simulink library "halin"  (R2021b)
settings: Solver=VariableStepAuto  StartTime=0.0  StopTime=10.0  RelTol=1e-3
undefined symbols (not defined in the file): KHAL_CAN1ABM1E2E_flg, KHAL_CAN1EPB1E2E_flg, KHAL_CAN1EPS1E2E_flg, KHAL_CAN1ESC1E2E_flg, KHAL_CAN1ESC5E2E_flg, KHAL_CAN3BMS1E2E_flg, KHAL_CAN3BMS6E2E_flg, KHAL_CAN3CCU1E2E_flg, KHAL_CAN3CCU2E2E_flg, KHAL_CAN3MCUBF1E2E_flg, KHAL_CAN3MCUBR1E2E_flg, KHAL_CAN3MCUNF1E2E_flg, KHAL_CAN3MCUNR1E2E_flg, KHAL_CAN3Shifter1E2E_flg, KHAL_CAN3Shifter2E2E_flg, KHAL_CAN6FCM2E2E_flg, KHAL_CAN6FCM4E2E_flg, TRUE
libraries: simulink x791, FVT_lib x214, hcu_lib x58
(part 14 of 25)

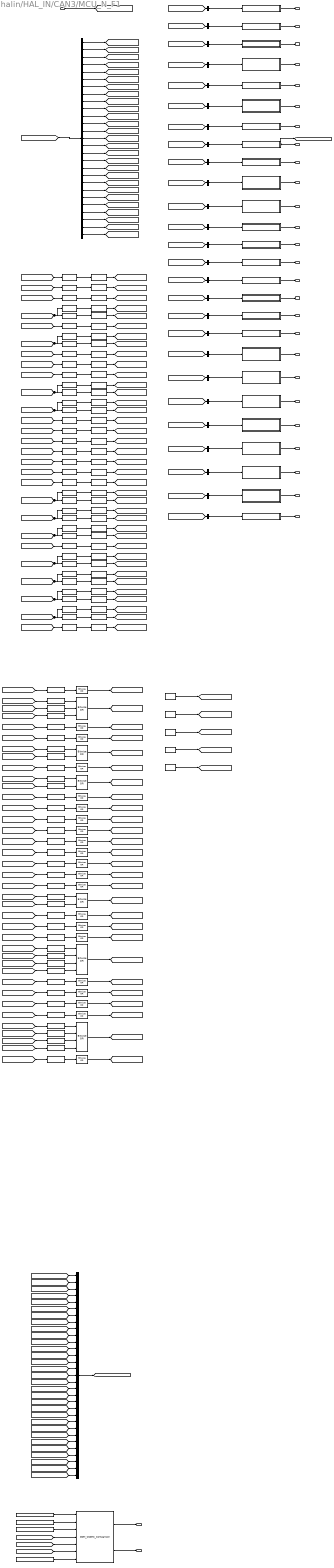
== system halin/HAL_IN/CAN3/MCU_N_F1 ==
  DT_CAN3_SG_MCU_N_F1 : Inport
  0x95 : Constant  Value=0x95
  0xF9 : Constant  Value=0xF9
  BitwiseAND{,1..37} (38 alike) : simulink/Logic and Bit Operations/Bitwise Operator  logicop=AND  UseBitMask=on  BitMask=0xFF  BitMaskRealWorld=Stored Integer
  BitwiseOR{,2..3,5,7..15,17..19,21..24,26} (21 alike) : simulink/Logic and Bit Operations/Bitwise Operator  logicop=OR  UseBitMask=off  BitMask=bin2dec('11011001')  BitMaskRealWorld=Stored Integer
  BitwiseOR1 : simulink/Logic and Bit Operations/Bitwise Operator  logicop=OR  UseBitMask=off  NumInputPorts=3  BitMask=bin2dec('11011001')  BitMaskRealWorld=Stored Integer
  BitwiseOR16 : simulink/Logic and Bit Operations/Bitwise Operator  logicop=OR  UseBitMask=off  NumInputPorts=2  BitMask=bin2dec('11011001')  BitMaskRealWorld=Stored Integer
  BitwiseOR20 : simulink/Logic and Bit Operations/Bitwise Operator  logicop=OR  UseBitMask=off  NumInputPorts=4  BitMask=bin2dec('11011001')  BitMaskRealWorld=Stored Integer
  BitwiseOR25 : simulink/Logic and Bit Operations/Bitwise Operator  logicop=OR  UseBitMask=off  NumInputPorts=4  BitMask=bin2dec('11011001')  BitMaskRealWorld=Stored Integer
  BitwiseOR4 : simulink/Logic and Bit Operations/Bitwise Operator  logicop=OR  UseBitMask=off  NumInputPorts=2  BitMask=bin2dec('11011001')  BitMaskRealWorld=Stored Integer
  BitwiseOR6 : simulink/Logic and Bit Operations/Bitwise Operator  logicop=OR  UseBitMask=off  NumInputPorts=2  BitMask=bin2dec('11011001')  BitMaskRealWorld=Stored Integer
  DDM_CS&RC_Comparison : FVT_lib/hal/DDM_CS&RC_Comparison  MsgCycleTime=100
  Data Type Conversion{,1..37} (38 alike) : DataTypeConversion  OutDataTypeStr=uint8
  FrActvDmpDisabStaNidec : Subsystem
  FrEDUDrtStaNidec : Subsystem
  FrEDUOpratingStaNidec : Subsystem
  FrEDURealTMTqNidec : Subsystem
  FrEDURotateDirctionNidec : Subsystem
  FrEDUTqReqFbkNidec : Subsystem
  FrMCU1ChksumNidec : Subsystem
  FrMCU1RolCntNidec : Subsystem
  FrMCUBATNidec : Subsystem
  FrMCUDCBusCurrNidec : Subsystem
  FrMCUDCBusVoltNidec : Subsystem
  FrMCUDischrgStaNidec : Subsystem
  FrMCUEnaStaNidec : Subsystem
  FrMCUErrNidec : Subsystem
  FrMCUIGNstaNidec : Subsystem
  FrMCUReady4PreNidec : Subsystem
  FrMCUReadyNidec : Subsystem
  FrMCUSysStaNidec : Subsystem
  FrMCUTempNidec : Subsystem
  FrMotorAvailTqNidec : Subsystem
  FrRegenAvailTqNidec : Subsystem
  FrTMSpdNidec : Subsystem
  FrTMTempNidec : Subsystem
  FrTMidNidec : Subsystem
  FrTMiqNidec : Subsystem
  KHAL_CAN3MCUNF1E2E_flg : Constant  Value=KHAL_CAN3MCUNF1E2E_flg
  LeftShift : ArithShift  BitShiftNumber=1  BitShiftDirection=Left
  LeftShift1 : ArithShift  BitShiftNumber=2  BitShiftDirection=Left
  LeftShift{4,6,9..11,13,15} (7 alike) : ArithShift  BitShiftDirection=Left
  LeftShift12 : ArithShift  BitShiftNumber=3  BitShiftDirection=Left
  LeftShift14 : ArithShift  BitShiftNumber=1  BitShiftDirection=Left
  LeftShift2 : ArithShift  BitShiftNumber=5  BitShiftDirection=Left
  LeftShift3 : ArithShift  BitShiftNumber=6  BitShiftDirection=Left
  LeftShift5 : ArithShift  BitShiftNumber=4  BitShiftDirection=Left
  LeftShift7 : ArithShift  BitShiftNumber=3  BitShiftDirection=Left
  LeftShift8 : ArithShift  BitShiftNumber=4  BitShiftDirection=Left
  MCUWarnFNidec : Subsystem
  MessageRollingCounter : FVT_lib/hal/MessageRollingCounter  CounterMAX=14  task_time_ms=5  msg_time_ms=100
  Mux : Mux  Inputs=31
  RightShift{,2,4,6,10,14,16,18,20} (9 alike) : ArithShift  BitShiftNumber=8
  RightShift{1,3,5,7,11,15,17,19,21} (9 alike) : ArithShift
  RightShift12 : ArithShift  BitShiftNumber=4
  RightShift13 : ArithShift  BitShiftNumber=-4
  RightShift8 : ArithShift  BitShiftNumber=1
  RightShift9 : ArithShift  BitShiftNumber=-7
  bus_selector : BusSelector  OutputSignals=CAN3_Fr_ActvDmpDisabSta_Nidec,CAN3_Fr_EDUDrtSta_Nidec,CAN3_Fr_EDUOpratingSta_Nidec,CAN3_Fr_EDURealTMTq_Nidec,CAN3_Fr_EDURotateDirction_Nidec,CAN3_Fr_EDUTqReqFbk_Nidec,CAN3_Fr_MCU1Chksum_Nidec,CAN3_Fr_MCU1RolCnt_Nidec,CAN3_Fr_MCUBAT_Nidec,CAN3_Fr_MCUDCBusCurr_Nidec,CAN3_Fr_MCUDCBusVolt_Nidec,CAN3_Fr_MCUDischrgSta_Nidec,CAN3_Fr_MCUEnaSta_Nidec,CAN3_Fr_MCUErr_Nidec,CAN3_Fr_MCUIGN_sta_Nidec,CAN3_Fr_MCUReady4Pre_Nidec,CAN3_Fr_MCUReady_Nidec,CAN3_Fr_MCUSysSta_Nidec,CAN3_Fr_MCUTemp_Nidec,CAN3_Fr_MotorAvailTq_Nidec,CAN3_Fr_RegenAvailTq_Nidec,CAN3_Fr_Reserved_bits_Nidec,CAN3_Fr_TMSpd_Nidec,CAN3_Fr_TMTemp_Nidec,CAN3_Fr_TMid_Nidec,CAN3_Fr_TMiq_Nidec,CAN3_MCUWarn_F_Nidec
  bus_selector1 : BusSelector  OutputSignals=CAN3_Fr_ActvDmpDisabSta_Nidec
  bus_selector10 : BusSelector  OutputSignals=CAN3_Fr_MCUDCBusCurr_Nidec
  bus_selector11 : BusSelector  OutputSignals=CAN3_Fr_MCUDCBusVolt_Nidec
  bus_selector12 : BusSelector  OutputSignals=CAN3_Fr_MCUDischrgSta_Nidec
  bus_selector13 : BusSelector  OutputSignals=CAN3_Fr_MCUEnaSta_Nidec
  bus_selector14 : BusSelector  OutputSignals=CAN3_Fr_MCUErr_Nidec
  bus_selector15 : BusSelector  OutputSignals=CAN3_Fr_MCUIGN_sta_Nidec
  bus_selector16 : BusSelector  OutputSignals=CAN3_Fr_MCUReady4Pre_Nidec
  bus_selector17 : BusSelector  OutputSignals=CAN3_Fr_MCUReady_Nidec
  bus_selector18 : BusSelector  OutputSignals=CAN3_Fr_MCUSysSta_Nidec
  bus_selector19 : BusSelector  OutputSignals=CAN3_Fr_MCUTemp_Nidec
  bus_selector2 : BusSelector  OutputSignals=CAN3_Fr_EDUDrtSta_Nidec
  bus_selector20 : BusSelector  OutputSignals=CAN3_Fr_MotorAvailTq_Nidec
  bus_selector21 : BusSelector  OutputSignals=CAN3_Fr_RegenAvailTq_Nidec
  bus_selector22 : BusSelector  OutputSignals=CAN3_Fr_TMSpd_Nidec
  bus_selector23 : BusSelector  OutputSignals=CAN3_Fr_TMTemp_Nidec
  bus_selector24 : BusSelector  OutputSignals=CAN3_Fr_TMid_Nidec
  bus_selector25 : BusSelector  OutputSignals=CAN3_Fr_TMiq_Nidec
  bus_selector26 : BusSelector  OutputSignals=CAN3_MCUWarn_F_Nidec
  bus_selector3 : BusSelector  OutputSignals=CAN3_Fr_EDUOpratingSta_Nidec
  bus_selector4 : BusSelector  OutputSignals=CAN3_Fr_EDURealTMTq_Nidec
  bus_selector5 : BusSelector  OutputSignals=CAN3_Fr_EDURotateDirction_Nidec
  bus_selector6 : BusSelector  OutputSignals=CAN3_Fr_EDUTqReqFbk_Nidec
  bus_selector7 : BusSelector  OutputSignals=CAN3_Fr_MCU1Chksum_Nidec
  bus_selector8 : BusSelector  OutputSignals=CAN3_Fr_MCU1RolCnt_Nidec
  bus_selector9 : BusSelector  OutputSignals=CAN3_Fr_MCUBAT_Nidec
  constant{,1..4} (5 alike) : Constant  Value=0x0  OutDataTypeStr=uint8
  VHAL_MCUNF1CSErr_flg : Outport
  VHAL_MCUNF1RCErr_flg : Outport  Port=2
  VHAL_FrActvDmpDisabStaNidec_flg : Outport  Port=3
  VHAL_FrEDUDrtStaNidec_flg : Outport  Port=4
  VHAL_FrEDUOpratingStaNidec_flg : Outport  Port=5
  VHAL_FrEDURealTMTqNidec_Nm : Outport  Port=6
  VHAL_FrEDURotateDirctionNidec_enum : Outport  Port=7
  VHAL_FrEDUTqReqFbkNidec_Nm : Outport  Port=8
  VHAL_FrMCU1ChksumNidec_enum : Outport  Port=9
  VHAL_FrMCU1RolCntNidec_enum : Outport  Port=10
  VHAL_FrMCUBATNidec_V : Outport  Port=11
  VHAL_FrMCUDCBusCurrNidec_A : Outport  Port=12
  VHAL_FrMCUDCBusVoltNidec_V : Outport  Port=13
  VHAL_FrMCUDischrgStaNidec_flg : Outport  Port=14
  VHAL_FrMCUEnaStaNidec_flg : Outport  Port=15
  VHAL_FrMCUErrNidec_enum : Outport  Port=16
  VHAL_FrMCUIGNstaNidec_flg : Outport  Port=17
  VHAL_FrMCUReady4PreNidec_flg : Outport  Port=18
  VHAL_FrMCUReadyNidec_flg : Outport  Port=19
  VHAL_FrMCUSysStaNidec_enum : Outport  Port=20
  VHAL_FrMCUTempNidec_C : Outport  Port=21
  VHAL_FrMotorAvailTqNidec_Nm : Outport  Port=22
  VHAL_FrRegenAvailTqNidec_Nm : Outport  Port=23
  VHAL_FrTMSpdNidec_rpm : Outport  Port=24
  VHAL_FrTMTempNidec_C : Outport  Port=25
  VHAL_FrTMidNidec_A : Outport  Port=26
  VHAL_FrTMiqNidec_A : Outport  Port=27
  VHAL_MCUWarnFNidec_enum : Outport  Port=28
  wires:
  DT_CAN3_SG_MCU_N_F1/1 -> [DT_CAN3_SG_MCU_N_F1]
  [DT_CAN3_SG_MCU_N_F1] -> bus_selector/1
  bus_selector/1 -> [CAN3_Fr_ActvDmpDisabSta_Nidec]  "<CAN3_Fr_ActvDmpDisabSta_Nidec>"
  [CAN3_Fr_ActvDmpDisabSta_Nidec] -> LeftShift/1
  LeftShift/1 -> BitwiseAND/1
  BitwiseAND/1 -> [Byte_25_CAN3_Fr_ActvDmpDisabSta_Nidec]
  bus_selector/2 -> [CAN3_Fr_EDUDrtSta_Nidec]  "<CAN3_Fr_EDUDrtSta_Nidec>"
  [CAN3_Fr_EDUDrtSta_Nidec] -> LeftShift1/1
  LeftShift1/1 -> BitwiseAND1/1
  BitwiseAND1/1 -> [Byte_25_CAN3_Fr_EDUDrtSta_Nidec]
  bus_selector/3 -> [CAN3_Fr_EDUOpratingSta_Nidec]  "<CAN3_Fr_EDUOpratingSta_Nidec>"
  [CAN3_Fr_EDUOpratingSta_Nidec] -> LeftShift2/1
  LeftShift2/1 -> BitwiseAND2/1
  BitwiseAND2/1 -> [Byte_30_CAN3_Fr_EDUOpratingSta_Nidec]
  bus_selector/4 -> [CAN3_Fr_EDURealTMTq_Nidec]  "<CAN3_Fr_EDURealTMTq_Nidec>"
  [CAN3_Fr_EDURealTMTq_Nidec] -> RightShift/1, RightShift1/1
  RightShift/1 -> BitwiseAND3/1
  BitwiseAND3/1 -> [Byte_28_CAN3_Fr_EDURealTMTq_Nidec]
  RightShift1/1 -> BitwiseAND4/1
  BitwiseAND4/1 -> [Byte_29_CAN3_Fr_EDURealTMTq_Nidec]
  bus_selector/5 -> [CAN3_Fr_EDURotateDirction_Nidec]  "<CAN3_Fr_EDURotateDirction_Nidec>"
  [CAN3_Fr_EDURotateDirction_Nidec] -> LeftShift3/1
  LeftShift3/1 -> BitwiseAND5/1
  BitwiseAND5/1 -> [Byte_30_CAN3_Fr_EDURotateDirction_Nidec]
  bus_selector/6 -> [CAN3_Fr_EDUTqReqFbk_Nidec]  "<CAN3_Fr_EDUTqReqFbk_Nidec>"
  [CAN3_Fr_EDUTqReqFbk_Nidec] -> RightShift2/1, RightShift3/1
  RightShift2/1 -> BitwiseAND6/1
  BitwiseAND6/1 -> [Byte_30_CAN3_Fr_EDUTqReqFbk_Nidec]
  RightShift3/1 -> BitwiseAND7/1
  BitwiseAND7/1 -> [Byte_31_CAN3_Fr_EDUTqReqFbk_Nidec]
  bus_selector/7 -> [CAN3_Fr_MCU1Chksum_Nidec]  "<CAN3_Fr_MCU1Chksum_Nidec>"
  [CAN3_Fr_MCU1Chksum_Nidec] -> LeftShift4/1
  LeftShift4/1 -> BitwiseAND8/1
  BitwiseAND8/1 -> [Byte_0_CAN3_Fr_MCU1Chksum_Nidec]
  bus_selector/8 -> [CAN3_Fr_MCU1RolCnt_Nidec]  "<CAN3_Fr_MCU1RolCnt_Nidec>"
  [CAN3_Fr_MCU1RolCnt_Nidec] -> LeftShift5/1
  LeftShift5/1 -> BitwiseAND9/1
  BitwiseAND9/1 -> [Byte_1_CAN3_Fr_MCU1RolCnt_Nidec]
  bus_selector/9 -> [CAN3_Fr_MCUBAT_Nidec]  "<CAN3_Fr_MCUBAT_Nidec>"
  [CAN3_Fr_MCUBAT_Nidec] -> LeftShift6/1
  LeftShift6/1 -> BitwiseAND10/1
  BitwiseAND10/1 -> [Byte_8_CAN3_Fr_MCUBAT_Nidec]
  bus_selector/10 -> [CAN3_Fr_MCUDCBusCurr_Nidec]  "<CAN3_Fr_MCUDCBusCurr_Nidec>"
  [CAN3_Fr_MCUDCBusCurr_Nidec] -> RightShift4/1, RightShift5/1
  RightShift4/1 -> BitwiseAND11/1
  BitwiseAND11/1 -> [Byte_21_CAN3_Fr_MCUDCBusCurr_Nidec]
  RightShift5/1 -> BitwiseAND12/1
  BitwiseAND12/1 -> [Byte_22_CAN3_Fr_MCUDCBusCurr_Nidec]
  bus_selector/11 -> [CAN3_Fr_MCUDCBusVolt_Nidec]  "<CAN3_Fr_MCUDCBusVolt_Nidec>"
  [CAN3_Fr_MCUDCBusVolt_Nidec] -> RightShift6/1, RightShift7/1
  RightShift6/1 -> BitwiseAND13/1
  BitwiseAND13/1 -> [Byte_23_CAN3_Fr_MCUDCBusVolt_Nidec]
  RightShift7/1 -> BitwiseAND14/1
  BitwiseAND14/1 -> [Byte_24_CAN3_Fr_MCUDCBusVolt_Nidec]
  bus_selector/12 -> [CAN3_Fr_MCUDischrgSta_Nidec]  "<CAN3_Fr_MCUDischrgSta_Nidec>"
  [CAN3_Fr_MCUDischrgSta_Nidec] -> LeftShift7/1
  LeftShift7/1 -> BitwiseAND15/1
  BitwiseAND15/1 -> [Byte_25_CAN3_Fr_MCUDischrgSta_Nidec]
  bus_selector/13 -> [CAN3_Fr_MCUEnaSta_Nidec]  "<CAN3_Fr_MCUEnaSta_Nidec>"
  [CAN3_Fr_MCUEnaSta_Nidec] -> LeftShift8/1
  LeftShift8/1 -> BitwiseAND16/1
  BitwiseAND16/1 -> [Byte_30_CAN3_Fr_MCUEnaSta_Nidec]
  bus_selector/14 -> [CAN3_Fr_MCUErr_Nidec]  "<CAN3_Fr_MCUErr_Nidec>"
  [CAN3_Fr_MCUErr_Nidec] -> LeftShift9/1
  LeftShift9/1 -> BitwiseAND17/1
  BitwiseAND17/1 -> [Byte_17_CAN3_Fr_MCUErr_Nidec]
  bus_selector/15 -> [CAN3_Fr_MCUIGN_sta_Nidec]  "<CAN3_Fr_MCUIGN_sta_Nidec>"
  [CAN3_Fr_MCUIGN_sta_Nidec] -> LeftShift10/1
  LeftShift10/1 -> BitwiseAND18/1
  BitwiseAND18/1 -> [Byte_9_CAN3_Fr_MCUIGN_sta_Nidec]
  bus_selector/16 -> [CAN3_Fr_MCUReady4Pre_Nidec]  "<CAN3_Fr_MCUReady4Pre_Nidec>"
  [CAN3_Fr_MCUReady4Pre_Nidec] -> LeftShift11/1
  LeftShift11/1 -> BitwiseAND19/1
  BitwiseAND19/1 -> [Byte_25_CAN3_Fr_MCUReady4Pre_Nidec]
  bus_selector/17 -> [CAN3_Fr_MCUReady_Nidec]  "<CAN3_Fr_MCUReady_Nidec>"
  [CAN3_Fr_MCUReady_Nidec] -> LeftShift12/1
  LeftShift12/1 -> BitwiseAND20/1
  BitwiseAND20/1 -> [Byte_1_CAN3_Fr_MCUReady_Nidec]
  bus_selector/18 -> [CAN3_Fr_MCUSysSta_Nidec]  "<CAN3_Fr_MCUSysSta_Nidec>"
  [CAN3_Fr_MCUSysSta_Nidec] -> LeftShift13/1
  LeftShift13/1 -> BitwiseAND21/1
  BitwiseAND21/1 -> [Byte_7_CAN3_Fr_MCUSysSta_Nidec]
  bus_selector/19 -> [CAN3_Fr_MCUTemp_Nidec]  "<CAN3_Fr_MCUTemp_Nidec>"
  [CAN3_Fr_MCUTemp_Nidec] -> RightShift8/1, RightShift9/1
  RightShift8/1 -> BitwiseAND22/1
  BitwiseAND22/1 -> [Byte_20_CAN3_Fr_MCUTemp_Nidec]
  RightShift9/1 -> BitwiseAND23/1
  BitwiseAND23/1 -> [Byte_21_CAN3_Fr_MCUTemp_Nidec]
  bus_selector/20 -> [CAN3_Fr_MotorAvailTq_Nidec]  "<CAN3_Fr_MotorAvailTq_Nidec>"
  [CAN3_Fr_MotorAvailTq_Nidec] -> RightShift10/1, RightShift11/1
  RightShift10/1 -> BitwiseAND24/1
  BitwiseAND24/1 -> [Byte_11_CAN3_Fr_MotorAvailTq_Nidec]
  RightShift11/1 -> BitwiseAND25/1
  BitwiseAND25/1 -> [Byte_12_CAN3_Fr_MotorAvailTq_Nidec]
  bus_selector/21 -> [CAN3_Fr_RegenAvailTq_Nidec]  "<CAN3_Fr_RegenAvailTq_Nidec>"
  [CAN3_Fr_RegenAvailTq_Nidec] -> RightShift12/1, RightShift13/1
  RightShift12/1 -> BitwiseAND26/1
  BitwiseAND26/1 -> [Byte_10_CAN3_Fr_RegenAvailTq_Nidec]
  RightShift13/1 -> BitwiseAND27/1
  BitwiseAND27/1 -> [Byte_11_CAN3_Fr_RegenAvailTq_Nidec]
  bus_selector/22 -> [CAN3_Fr_Reserved_bits_Nidec]  "<CAN3_Fr_Reserved_bits_Nidec>"
  [CAN3_Fr_Reserved_bits_Nidec] -> LeftShift14/1
  LeftShift14/1 -> BitwiseAND28/1
  BitwiseAND28/1 -> [Byte_9_CAN3_Fr_Reserved_bits_Nidec]
  bus_selector/23 -> [CAN3_Fr_TMSpd_Nidec]  "<CAN3_Fr_TMSpd_Nidec>"
  [CAN3_Fr_TMSpd_Nidec] -> RightShift14/1, RightShift15/1
  RightShift14/1 -> BitwiseAND29/1
  BitwiseAND29/1 -> [Byte_26_CAN3_Fr_TMSpd_Nidec]
  RightShift15/1 -> BitwiseAND30/1
  BitwiseAND30/1 -> [Byte_27_CAN3_Fr_TMSpd_Nidec]
  bus_selector/24 -> [CAN3_Fr_TMTemp_Nidec]  "<CAN3_Fr_TMTemp_Nidec>"
  [CAN3_Fr_TMTemp_Nidec] -> RightShift16/1, RightShift17/1
  RightShift16/1 -> BitwiseAND31/1
  BitwiseAND31/1 -> [Byte_18_CAN3_Fr_TMTemp_Nidec]
  RightShift17/1 -> BitwiseAND32/1
  BitwiseAND32/1 -> [Byte_19_CAN3_Fr_TMTemp_Nidec]
  bus_selector/25 -> [CAN3_Fr_TMid_Nidec]  "<CAN3_Fr_TMid_Nidec>"
  [CAN3_Fr_TMid_Nidec] -> RightShift18/1, RightShift19/1
  RightShift18/1 -> BitwiseAND33/1
  BitwiseAND33/1 -> [Byte_15_CAN3_Fr_TMid_Nidec]
  RightShift19/1 -> BitwiseAND34/1
  BitwiseAND34/1 -> [Byte_16_CAN3_Fr_TMid_Nidec]
  bus_selector/26 -> [CAN3_Fr_TMiq_Nidec]  "<CAN3_Fr_TMiq_Nidec>"
  [CAN3_Fr_TMiq_Nidec] -> RightShift20/1, RightShift21/1
  RightShift20/1 -> BitwiseAND35/1
  BitwiseAND35/1 -> [Byte_13_CAN3_Fr_TMiq_Nidec]
  RightShift21/1 -> BitwiseAND36/1
  BitwiseAND36/1 -> [Byte_14_CAN3_Fr_TMiq_Nidec]
  bus_selector/27 -> [CAN3_MCUWarn_F_Nidec]  "<CAN3_MCUWarn_F_Nidec>"
  [CAN3_MCUWarn_F_Nidec] -> LeftShift15/1
  LeftShift15/1 -> BitwiseAND37/1
  BitwiseAND37/1 -> [Byte_1_CAN3_MCUWarn_F_Nidec]
  Data Type Conversion/1 -> BitwiseOR/1
  [Byte_0_CAN3_Fr_MCU1Chksum_Nidec] -> Data Type Conversion/1
  BitwiseOR/1 -> [Byte_0]
  Data Type Conversion1/1 -> BitwiseOR1/1
  [Byte_1_CAN3_Fr_MCU1RolCnt_Nidec] -> Data Type Conversion1/1
  Data Type Conversion2/1 -> BitwiseOR1/2
  [Byte_1_CAN3_Fr_MCUReady_Nidec] -> Data Type Conversion2/1
  Data Type Conversion3/1 -> BitwiseOR1/3
  [Byte_1_CAN3_MCUWarn_F_Nidec] -> Data Type Conversion3/1
  BitwiseOR1/1 -> [Byte_1]
  constant/1 -> [Byte_2]
  constant1/1 -> [Byte_3]
  constant2/1 -> [Byte_4]
  constant3/1 -> [Byte_5]
  constant4/1 -> [Byte_6]
  Data Type Conversion4/1 -> BitwiseOR2/1
  [Byte_7_CAN3_Fr_MCUSysSta_Nidec] -> Data Type Conversion4/1
  BitwiseOR2/1 -> [Byte_7]
  Data Type Conversion5/1 -> BitwiseOR3/1
  [Byte_8_CAN3_Fr_MCUBAT_Nidec] -> Data Type Conversion5/1
  BitwiseOR3/1 -> [Byte_8]
  Data Type Conversion6/1 -> BitwiseOR4/1
  [Byte_9_CAN3_Fr_MCUIGN_sta_Nidec] -> Data Type Conversion6/1
  Data Type Conversion7/1 -> BitwiseOR4/2
  [Byte_9_CAN3_Fr_Reserved_bits_Nidec] -> Data Type Conversion7/1
  BitwiseOR4/1 -> [Byte_9]
  Data Type Conversion8/1 -> BitwiseOR5/1
  [Byte_10_CAN3_Fr_RegenAvailTq_Nidec] -> Data Type Conversion8/1
  BitwiseOR5/1 -> [Byte_10]
  Data Type Conversion9/1 -> BitwiseOR6/1
  [Byte_11_CAN3_Fr_MotorAvailTq_Nidec] -> Data Type Conversion9/1
  Data Type Conversion10/1 -> BitwiseOR6/2
  [Byte_11_CAN3_Fr_RegenAvailTq_Nidec] -> Data Type Conversion10/1
  BitwiseOR6/1 -> [Byte_11]
  Data Type Conversion11/1 -> BitwiseOR7/1
  [Byte_12_CAN3_Fr_MotorAvailTq_Nidec] -> Data Type Conversion11/1
  BitwiseOR7/1 -> [Byte_12]
  Data Type Conversion12/1 -> BitwiseOR8/1
  [Byte_13_CAN3_Fr_TMiq_Nidec] -> Data Type Conversion12/1
  BitwiseOR8/1 -> [Byte_13]
  Data Type Conversion13/1 -> BitwiseOR9/1
  [Byte_14_CAN3_Fr_TMiq_Nidec] -> Data Type Conversion13/1
  BitwiseOR9/1 -> [Byte_14]
  Data Type Conversion14/1 -> BitwiseOR10/1
  [Byte_15_CAN3_Fr_TMid_Nidec] -> Data Type Conversion14/1
  BitwiseOR10/1 -> [Byte_15]
  Data Type Conversion15/1 -> BitwiseOR11/1
  [Byte_16_CAN3_Fr_TMid_Nidec] -> Data Type Conversion15/1
  BitwiseOR11/1 -> [Byte_16]
  Data Type Conversion16/1 -> BitwiseOR12/1
  [Byte_17_CAN3_Fr_MCUErr_Nidec] -> Data Type Conversion16/1
  BitwiseOR12/1 -> [Byte_17]
  Data Type Conversion17/1 -> BitwiseOR13/1
  [Byte_18_CAN3_Fr_TMTemp_Nidec] -> Data Type Conversion17/1
  BitwiseOR13/1 -> [Byte_18]
  Data Type Conversion18/1 -> BitwiseOR14/1
  [Byte_19_CAN3_Fr_TMTemp_Nidec] -> Data Type Conversion18/1
  BitwiseOR14/1 -> [Byte_19]
  Data Type Conversion19/1 -> BitwiseOR15/1
  [Byte_20_CAN3_Fr_MCUTemp_Nidec] -> Data Type Conversion19/1
  BitwiseOR15/1 -> [Byte_20]
  Data Type Conversion20/1 -> BitwiseOR16/1
  [Byte_21_CAN3_Fr_MCUDCBusCurr_Nidec] -> Data Type Conversion20/1
  Data Type Conversion21/1 -> BitwiseOR16/2
  [Byte_21_CAN3_Fr_MCUTemp_Nidec] -> Data Type Conversion21/1
  BitwiseOR16/1 -> [Byte_21]
  Data Type Conversion22/1 -> BitwiseOR17/1
  [Byte_22_CAN3_Fr_MCUDCBusCurr_Nidec] -> Data Type Conversion22/1
  BitwiseOR17/1 -> [Byte_22]
  Data Type Conversion23/1 -> BitwiseOR18/1
  [Byte_23_CAN3_Fr_MCUDCBusVolt_Nidec] -> Data Type Conversion23/1
  BitwiseOR18/1 -> [Byte_23]
  Data Type Conversion24/1 -> BitwiseOR19/1
  [Byte_24_CAN3_Fr_MCUDCBusVolt_Nidec] -> Data Type Conversion24/1
  BitwiseOR19/1 -> [Byte_24]
  Data Type Conversion25/1 -> BitwiseOR20/1
  [Byte_25_CAN3_Fr_ActvDmpDisabSta_Nidec] -> Data Type Conversion25/1
  Data Type Conversion26/1 -> BitwiseOR20/2
  [Byte_25_CAN3_Fr_EDUDrtSta_Nidec] -> Data Type Conversion26/1
  Data Type Conversion27/1 -> BitwiseOR20/3
  [Byte_25_CAN3_Fr_MCUDischrgSta_Nidec] -> Data Type Conversion27/1
  Data Type Conversion28/1 -> BitwiseOR20/4
  [Byte_25_CAN3_Fr_MCUReady4Pre_Nidec] -> Data Type Conversion28/1
  BitwiseOR20/1 -> [Byte_25]
  Data Type Conversion29/1 -> BitwiseOR21/1
  [Byte_26_CAN3_Fr_TMSpd_Nidec] -> Data Type Conversion29/1
  BitwiseOR21/1 -> [Byte_26]
  Data Type Conversion30/1 -> BitwiseOR22/1
  [Byte_27_CAN3_Fr_TMSpd_Nidec] -> Data Type Conversion30/1
  BitwiseOR22/1 -> [Byte_27]
  Data Type Conversion31/1 -> BitwiseOR23/1
  [Byte_28_CAN3_Fr_EDURealTMTq_Nidec] -> Data Type Conversion31/1
  BitwiseOR23/1 -> [Byte_28]
  Data Type Conversion32/1 -> BitwiseOR24/1
  [Byte_29_CAN3_Fr_EDURealTMTq_Nidec] -> Data Type Conversion32/1
  BitwiseOR24/1 -> [Byte_29]
  Data Type Conversion33/1 -> BitwiseOR25/1
  [Byte_30_CAN3_Fr_EDUOpratingSta_Nidec] -> Data Type Conversion33/1
  Data Type Conversion34/1 -> BitwiseOR25/2
  [Byte_30_CAN3_Fr_EDURotateDirction_Nidec] -> Data Type Conversion34/1
  Data Type Conversion35/1 -> BitwiseOR25/3
  [Byte_30_CAN3_Fr_EDUTqReqFbk_Nidec] -> Data Type Conversion35/1
  Data Type Conversion36/1 -> BitwiseOR25/4
  [Byte_30_CAN3_Fr_MCUEnaSta_Nidec] -> Data Type Conversion36/1
  BitwiseOR25/1 -> [Byte_30]
  Data Type Conversion37/1 -> BitwiseOR26/1
  [Byte_31_CAN3_Fr_EDUTqReqFbk_Nidec] -> Data Type Conversion37/1
  BitwiseOR26/1 -> [Byte_31]
  [Byte_1] -> Mux/1
  [Byte_2] -> Mux/2
  [Byte_3] -> Mux/3
  [Byte_4] -> Mux/4
  [Byte_5] -> Mux/5
  [Byte_6] -> Mux/6
  [Byte_7] -> Mux/7
  [Byte_8] -> Mux/8
  [Byte_9] -> Mux/9
  [Byte_10] -> Mux/10
  [Byte_11] -> Mux/11
  [Byte_12] -> Mux/12
  [Byte_13] -> Mux/13
  [Byte_14] -> Mux/14
  [Byte_15] -> Mux/15
  [Byte_16] -> Mux/16
  [Byte_17] -> Mux/17
  [Byte_18] -> Mux/18
  [Byte_19] -> Mux/19
  [Byte_20] -> Mux/20
  [Byte_21] -> Mux/21
  [Byte_22] -> Mux/22
  [Byte_23] -> Mux/23
  [Byte_24] -> Mux/24
  [Byte_25] -> Mux/25
  [Byte_26] -> Mux/26
  [Byte_27] -> Mux/27
  [Byte_28] -> Mux/28
  [Byte_29] -> Mux/29
  [Byte_30] -> Mux/30
  [Byte_31] -> Mux/31
  Mux/1 -> [VHAL_CAN3MCUNF1noCS_raw]
  KHAL_CAN3MCUNF1E2E_flg/1 -> DDM_CS&RC_Comparison/1
  0xF9/1 -> DDM_CS&RC_Comparison/2
  0x95/1 -> DDM_CS&RC_Comparison/3
  [VHAL_CAN3MCUNF1noCS_raw] -> DDM_CS&RC_Comparison/4
  [Byte_0] -> DDM_CS&RC_Comparison/5
  [RC_ECU] -> DDM_CS&RC_Comparison/6
  MessageRollingCounter/1 -> DDM_CS&RC_Comparison/7
  DDM_CS&RC_Comparison/1 -> VHAL_MCUNF1CSErr_flg/1
  DDM_CS&RC_Comparison/2 -> VHAL_MCUNF1RCErr_flg/1
  [DT_CAN3_SG_MCU_N_F1] -> bus_selector1/1
  bus_selector1/1 -> FrActvDmpDisabStaNidec/1(Fr_ActvDmpDisabSta_Nidec)  "<CAN3_Fr_ActvDmpDisabSta_Nidec>"
  FrActvDmpDisabStaNidec/1(VHAL_FrActvDmpDisabStaNidec_flg) -> VHAL_FrActvDmpDisabStaNidec_flg/1
  [DT_CAN3_SG_MCU_N_F1] -> bus_selector2/1
  bus_selector2/1 -> FrEDUDrtStaNidec/1(Fr_EDUDrtSta_Nidec)  "<CAN3_Fr_EDUDrtSta_Nidec>"
  FrEDUDrtStaNidec/1(VHAL_FrEDUDrtStaNidec_flg) -> VHAL_FrEDUDrtStaNidec_flg/1
  [DT_CAN3_SG_MCU_N_F1] -> bus_selector3/1
  bus_selector3/1 -> FrEDUOpratingStaNidec/1(Fr_EDUOpratingSta_Nidec)  "<CAN3_Fr_EDUOpratingSta_Nidec>"
  FrEDUOpratingStaNidec/1(VHAL_FrEDUOpratingStaNidec_flg) -> VHAL_FrEDUOpratingStaNidec_flg/1
  [DT_CAN3_SG_MCU_N_F1] -> bus_selector4/1
  bus_selector4/1 -> FrEDURealTMTqNidec/1(Fr_EDURealTMTq_Nidec)  "<CAN3_Fr_EDURealTMTq_Nidec>"
  FrEDURealTMTqNidec/1(VHAL_FrEDURealTMTqNidec_Nm) -> VHAL_FrEDURealTMTqNidec_Nm/1
  [DT_CAN3_SG_MCU_N_F1] -> bus_selector5/1
  bus_selector5/1 -> FrEDURotateDirctionNidec/1(Fr_EDURotateDirction_Nidec)  "<CAN3_Fr_EDURotateDirction_Nidec>"
  FrEDURotateDirctionNidec/1(VHAL_FrEDURotateDirctionNidec_enum) -> VHAL_FrEDURotateDirctionNidec_enum/1
  [DT_CAN3_SG_MCU_N_F1] -> bus_selector6/1
  bus_selector6/1 -> FrEDUTqReqFbkNidec/1(Fr_EDUTqReqFbk_Nidec)  "<CAN3_Fr_EDUTqReqFbk_Nidec>"
  FrEDUTqReqFbkNidec/1(VHAL_FrEDUTqReqFbkNidec_Nm) -> VHAL_FrEDUTqReqFbkNidec_Nm/1
  [DT_CAN3_SG_MCU_N_F1] -> bus_selector7/1
  bus_selector7/1 -> FrMCU1ChksumNidec/1(Fr_MCU1Chksum_Nidec)  "<CAN3_Fr_MCU1Chksum_Nidec>"
  FrMCU1ChksumNidec/1(VHAL_FrMCU1ChksumNidec_enum) -> VHAL_FrMCU1ChksumNidec_enum/1
  [DT_CAN3_SG_MCU_N_F1] -> bus_selector8/1
  bus_selector8/1 -> FrMCU1RolCntNidec/1(Fr_MCU1RolCnt_Nidec)  "<CAN3_Fr_MCU1RolCnt_Nidec>"
  FrMCU1RolCntNidec/1(VHAL_FrMCU1RolCntNidec_enum) -> VHAL_FrMCU1RolCntNidec_enum/1, [RC_ECU]
  [DT_CAN3_SG_MCU_N_F1] -> bus_selector9/1
  bus_selector9/1 -> FrMCUBATNidec/1(Fr_MCUBAT_Nidec)  "<CAN3_Fr_MCUBAT_Nidec>"
  FrMCUBATNidec/1(VHAL_FrMCUBATNidec_V) -> VHAL_FrMCUBATNidec_V/1
  [DT_CAN3_SG_MCU_N_F1] -> bus_selector10/1
  bus_selector10/1 -> FrMCUDCBusCurrNidec/1(Fr_MCUDCBusCurr_Nidec)  "<CAN3_Fr_MCUDCBusCurr_Nidec>"
  FrMCUDCBusCurrNidec/1(VHAL_FrMCUDCBusCurrNidec_A) -> VHAL_FrMCUDCBusCurrNidec_A/1
  [DT_CAN3_SG_MCU_N_F1] -> bus_selector11/1
  bus_selector11/1 -> FrMCUDCBusVoltNidec/1(Fr_MCUDCBusVolt_Nidec)  "<CAN3_Fr_MCUDCBusVolt_Nidec>"
  FrMCUDCBusVoltNidec/1(VHAL_FrMCUDCBusVoltNidec_V) -> VHAL_FrMCUDCBusVoltNidec_V/1
  [DT_CAN3_SG_MCU_N_F1] -> bus_selector12/1
  bus_selector12/1 -> FrMCUDischrgStaNidec/1(Fr_MCUDischrgSta_Nidec)  "<CAN3_Fr_MCUDischrgSta_Nidec>"
  FrMCUDischrgStaNidec/1(VHAL_FrMCUDischrgStaNidec_flg) -> VHAL_FrMCUDischrgStaNidec_flg/1
  [DT_CAN3_SG_MCU_N_F1] -> bus_selector13/1
  bus_selector13/1 -> FrMCUEnaStaNidec/1(Fr_MCUEnaSta_Nidec)  "<CAN3_Fr_MCUEnaSta_Nidec>"
  FrMCUEnaStaNidec/1(VHAL_FrMCUEnaStaNidec_flg) -> VHAL_FrMCUEnaStaNidec_flg/1
  [DT_CAN3_SG_MCU_N_F1] -> bus_selector14/1
  bus_selector14/1 -> FrMCUErrNidec/1(Fr_MCUErr_Nidec)  "<CAN3_Fr_MCUErr_Nidec>"
  FrMCUErrNidec/1(VHAL_FrMCUErrNidec_enum) -> VHAL_FrMCUErrNidec_enum/1
  [DT_CAN3_SG_MCU_N_F1] -> bus_selector15/1
  bus_selector15/1 -> FrMCUIGNstaNidec/1(Fr_MCUIGN_sta_Nidec)  "<CAN3_Fr_MCUIGN_sta_Nidec>"
  FrMCUIGNstaNidec/1(VHAL_FrMCUIGNstaNidec_flg) -> VHAL_FrMCUIGNstaNidec_flg/1
  [DT_CAN3_SG_MCU_N_F1] -> bus_selector16/1
  bus_selector16/1 -> FrMCUReady4PreNidec/1(Fr_MCUReady4Pre_Nidec)  "<CAN3_Fr_MCUReady4Pre_Nidec>"
  FrMCUReady4PreNidec/1(VHAL_FrMCUReady4PreNidec_flg) -> VHAL_FrMCUReady4PreNidec_flg/1
  [DT_CAN3_SG_MCU_N_F1] -> bus_selector17/1
  bus_selector17/1 -> FrMCUReadyNidec/1(Fr_MCUReady_Nidec)  "<CAN3_Fr_MCUReady_Nidec>"
  FrMCUReadyNidec/1(VHAL_FrMCUReadyNidec_flg) -> VHAL_FrMCUReadyNidec_flg/1
  [DT_CAN3_SG_MCU_N_F1] -> bus_selector18/1
  bus_selector18/1 -> FrMCUSysStaNidec/1(Fr_MCUSysSta_Nidec)  "<CAN3_Fr_MCUSysSta_Nidec>"
  FrMCUSysStaNidec/1(VHAL_FrMCUSysStaNidec_enum) -> VHAL_FrMCUSysStaNidec_enum/1
  [DT_CAN3_SG_MCU_N_F1] -> bus_selector19/1
  bus_selector19/1 -> FrMCUTempNidec/1(Fr_MCUTemp_Nidec)  "<CAN3_Fr_MCUTemp_Nidec>"
  FrMCUTempNidec/1(VHAL_FrMCUTempNidec_C) -> VHAL_FrMCUTempNidec_C/1
  [DT_CAN3_SG_MCU_N_F1] -> bus_selector20/1
  bus_selector20/1 -> FrMotorAvailTqNidec/1(Fr_MotorAvailTq_Nidec)  "<CAN3_Fr_MotorAvailTq_Nidec>"
  FrMotorAvailTqNidec/1(VHAL_FrMotorAvailTqNidec_Nm) -> VHAL_FrMotorAvailTqNidec_Nm/1
  [DT_CAN3_SG_MCU_N_F1] -> bus_selector21/1
  bus_selector21/1 -> FrRegenAvailTqNidec/1(Fr_RegenAvailTq_Nidec)  "<CAN3_Fr_RegenAvailTq_Nidec>"
  FrRegenAvailTqNidec/1(VHAL_FrRegenAvailTqNidec_Nm) -> VHAL_FrRegenAvailTqNidec_Nm/1
  [DT_CAN3_SG_MCU_N_F1] -> bus_selector22/1
  bus_selector22/1 -> FrTMSpdNidec/1(Fr_TMSpd_Nidec)  "<CAN3_Fr_TMSpd_Nidec>"
  FrTMSpdNidec/1(VHAL_FrTMSpdNidec_rpm) -> VHAL_FrTMSpdNidec_rpm/1
  [DT_CAN3_SG_MCU_N_F1] -> bus_selector23/1
  bus_selector23/1 -> FrTMTempNidec/1(Fr_TMTemp_Nidec)  "<CAN3_Fr_TMTemp_Nidec>"
  FrTMTempNidec/1(VHAL_FrTMTempNidec_C) -> VHAL_FrTMTempNidec_C/1
  [DT_CAN3_SG_MCU_N_F1] -> bus_selector24/1
  bus_selector24/1 -> FrTMidNidec/1(Fr_TMid_Nidec)  "<CAN3_Fr_TMid_Nidec>"
  FrTMidNidec/1(VHAL_FrTMidNidec_A) -> VHAL_FrTMidNidec_A/1
  [DT_CAN3_SG_MCU_N_F1] -> bus_selector25/1
  bus_selector25/1 -> FrTMiqNidec/1(Fr_TMiq_Nidec)  "<CAN3_Fr_TMiq_Nidec>"
  FrTMiqNidec/1(VHAL_FrTMiqNidec_A) -> VHAL_FrTMiqNidec_A/1
  [DT_CAN3_SG_MCU_N_F1] -> bus_selector26/1
  bus_selector26/1 -> MCUWarnFNidec/1(MCUWarn_F_Nidec)  "<CAN3_MCUWarn_F_Nidec>"
  MCUWarnFNidec/1(VHAL_MCUWarnFNidec_enum) -> VHAL_MCUWarnFNidec_enum/1

== system halin/HAL_IN/CAN3/MCU_N_F2 ==
  DT_CAN3_SG_MCU_N_F2 : Inport
  FrCoolanttempReqNidec : Subsystem
  FrEOPSpdSetNidec : Subsystem
  FrFailcode1Nidec : Subsystem
  FrFailcode2Nidec : Subsystem
  FrFailcodehistory1Nidec : Subsystem
  FrFailcodehistory2Nidec : Subsystem
  FrLLCTempNidec : Subsystem
  FrLLCflowReqNidec : Subsystem
  FrMCUTempWarnNidec : Subsystem
  FrTMTempWarnNidec : Subsystem
  bus_selector : BusSelector  OutputSignals=CAN3_Fr_CoolanttempReq_Nidec
  bus_selector1 : BusSelector  OutputSignals=CAN3_Fr_EOP_SpdSet_Nidec
  bus_selector2 : BusSelector  OutputSignals=CAN3_Fr_Failcode1_Nidec
  bus_selector3 : BusSelector  OutputSignals=CAN3_Fr_Failcode2_Nidec
  bus_selector4 : BusSelector  OutputSignals=CAN3_Fr_Failcodehistory1_Nidec
  bus_selector5 : BusSelector  OutputSignals=CAN3_Fr_Failcodehistory2_Nidec
  bus_selector6 : BusSelector  OutputSignals=CAN3_Fr_LLCTemp_Nidec
  bus_selector7 : BusSelector  OutputSignals=CAN3_Fr_LLCflowReq_Nidec
  bus_selector8 : BusSelector  OutputSignals=CAN3_Fr_MCUTempWarn_Nidec
  bus_selector9 : BusSelector  OutputSignals=CAN3_Fr_TMTempWarn_Nidec
  VHAL_FrCoolanttempReqNidec_C : Outport
  VHAL_FrEOPSpdSetNidec_rpm : Outport  Port=2
  VHAL_FrFailcode1Nidec_enum : Outport  Port=3
  VHAL_FrFailcode2Nidec_enum : Outport  Port=4
  VHAL_FrFailcodehistory1Nidec_enum : Outport  Port=5
  VHAL_FrFailcodehistory2Nidec_enum : Outport  Port=6
  VHAL_FrLLCTempNidec_C : Outport  Port=7
  VHAL_FrLLCflowReqNidec_Lpmin : Outport  Port=8
  VHAL_FrMCUTempWarnNidec_enum : Outport  Port=9
  VHAL_FrTMTempWarnNidec_enum : Outport  Port=10
  wires:
  DT_CAN3_SG_MCU_N_F2/1 -> [DT_CAN3_SG_MCU_N_F2]
  [DT_CAN3_SG_MCU_N_F2] -> bus_selector/1
  bus_selector/1 -> FrCoolanttempReqNidec/1(Fr_CoolanttempReq_Nidec)  "<CAN3_Fr_CoolanttempReq_Nidec>"
  FrCoolanttempReqNidec/1(VHAL_FrCoolanttempReqNidec_C) -> VHAL_FrCoolanttempReqNidec_C/1
  [DT_CAN3_SG_MCU_N_F2] -> bus_selector1/1
  bus_selector1/1 -> FrEOPSpdSetNidec/1(Fr_EOP_SpdSet_Nidec)  "<CAN3_Fr_EOP_SpdSet_Nidec>"
  FrEOPSpdSetNidec/1(VHAL_FrEOPSpdSetNidec_rpm) -> VHAL_FrEOPSpdSetNidec_rpm/1
  [DT_CAN3_SG_MCU_N_F2] -> bus_selector2/1
  bus_selector2/1 -> FrFailcode1Nidec/1(Fr_Failcode1_Nidec)  "<CAN3_Fr_Failcode1_Nidec>"
  FrFailcode1Nidec/1(VHAL_FrFailcode1Nidec_enum) -> VHAL_FrFailcode1Nidec_enum/1
  [DT_CAN3_SG_MCU_N_F2] -> bus_selector3/1
  bus_selector3/1 -> FrFailcode2Nidec/1(Fr_Failcode2_Nidec)  "<CAN3_Fr_Failcode2_Nidec>"
  FrFailcode2Nidec/1(VHAL_FrFailcode2Nidec_enum) -> VHAL_FrFailcode2Nidec_enum/1
  [DT_CAN3_SG_MCU_N_F2] -> bus_selector4/1
  bus_selector4/1 -> FrFailcodehistory1Nidec/1(Fr_Failcodehistory1_Nidec)  "<CAN3_Fr_Failcodehistory1_Nidec>"
  FrFailcodehistory1Nidec/1(VHAL_FrFailcodehistory1Nidec_enum) -> VHAL_FrFailcodehistory1Nidec_enum/1
  [DT_CAN3_SG_MCU_N_F2] -> bus_selector5/1
  bus_selector5/1 -> FrFailcodehistory2Nidec/1(Fr_Failcodehistory2_Nidec)  "<CAN3_Fr_Failcodehistory2_Nidec>"
  FrFailcodehistory2Nidec/1(VHAL_FrFailcodehistory2Nidec_enum) -> VHAL_FrFailcodehistory2Nidec_enum/1
  [DT_CAN3_SG_MCU_N_F2] -> bus_selector6/1
  bus_selector6/1 -> FrLLCTempNidec/1(Fr_LLCTemp_Nidec)  "<CAN3_Fr_LLCTemp_Nidec>"
  FrLLCTempNidec/1(VHAL_FrLLCTempNidec_C) -> VHAL_FrLLCTempNidec_C/1
  [DT_CAN3_SG_MCU_N_F2] -> bus_selector7/1
  bus_selector7/1 -> FrLLCflowReqNidec/1(Fr_LLCflowReq_Nidec)  "<CAN3_Fr_LLCflowReq_Nidec>"
  FrLLCflowReqNidec/1(VHAL_FrLLCflowReqNidec_Lpmin) -> VHAL_FrLLCflowReqNidec_Lpmin/1
  [DT_CAN3_SG_MCU_N_F2] -> bus_selector8/1
  bus_selector8/1 -> FrMCUTempWarnNidec/1(Fr_MCUTempWarn_Nidec)  "<CAN3_Fr_MCUTempWarn_Nidec>"
  FrMCUTempWarnNidec/1(VHAL_FrMCUTempWarnNidec_enum) -> VHAL_FrMCUTempWarnNidec_enum/1
  [DT_CAN3_SG_MCU_N_F2] -> bus_selector9/1
  bus_selector9/1 -> FrTMTempWarnNidec/1(Fr_TMTempWarn_Nidec)  "<CAN3_Fr_TMTempWarn_Nidec>"
  FrTMTempWarnNidec/1(VHAL_FrTMTempWarnNidec_enum) -> VHAL_FrTMTempWarnNidec_enum/1

== system halin/HAL_IN/CAN3/MCU_N_F3 ==
  DT_CAN3_SG_MCU_N_F3 : Inport
  FrMCUHWVerNidec : Subsystem
  FrMCUSWVerNidec : Subsystem
  bus_selector : BusSelector  OutputSignals=CAN3_Fr_MCU_HW_Ver_Nidec
  bus_selector1 : BusSelector  OutputSignals=CAN3_Fr_MCU_SW_Ver_Nidec
  VHAL_FrMCUHWVerNidec_enum : Outport
  VHAL_FrMCUSWVerNidec_enum : Outport  Port=2
  wires:
  DT_CAN3_SG_MCU_N_F3/1 -> [DT_CAN3_SG_MCU_N_F3]
  [DT_CAN3_SG_MCU_N_F3] -> bus_selector/1
  bus_selector/1 -> FrMCUHWVerNidec/1(Fr_MCU_HW_Ver_Nidec)  "<CAN3_Fr_MCU_HW_Ver_Nidec>"
  FrMCUHWVerNidec/1(VHAL_FrMCUHWVerNidec_enum) -> VHAL_FrMCUHWVerNidec_enum/1
  [DT_CAN3_SG_MCU_N_F3] -> bus_selector1/1
  bus_selector1/1 -> FrMCUSWVerNidec/1(Fr_MCU_SW_Ver_Nidec)  "<CAN3_Fr_MCU_SW_Ver_Nidec>"
  FrMCUSWVerNidec/1(VHAL_FrMCUSWVerNidec_enum) -> VHAL_FrMCUSWVerNidec_enum/1
